simulink model "Fuzzy"  (R2024a)
settings: Solver=VariableStepAuto  StartTime=0.0  StopTime=200  RelTol=1e-3
libraries: fuzblock x1
settings Model: Creator=jyoti  LastModifiedBy=Admin

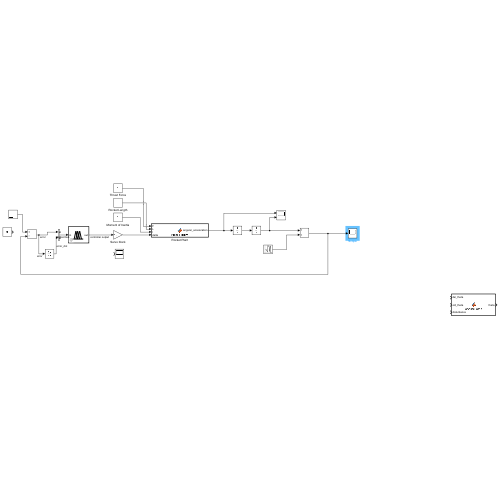
[thumbnail: Simulink's stored preview of the top-level diagram]
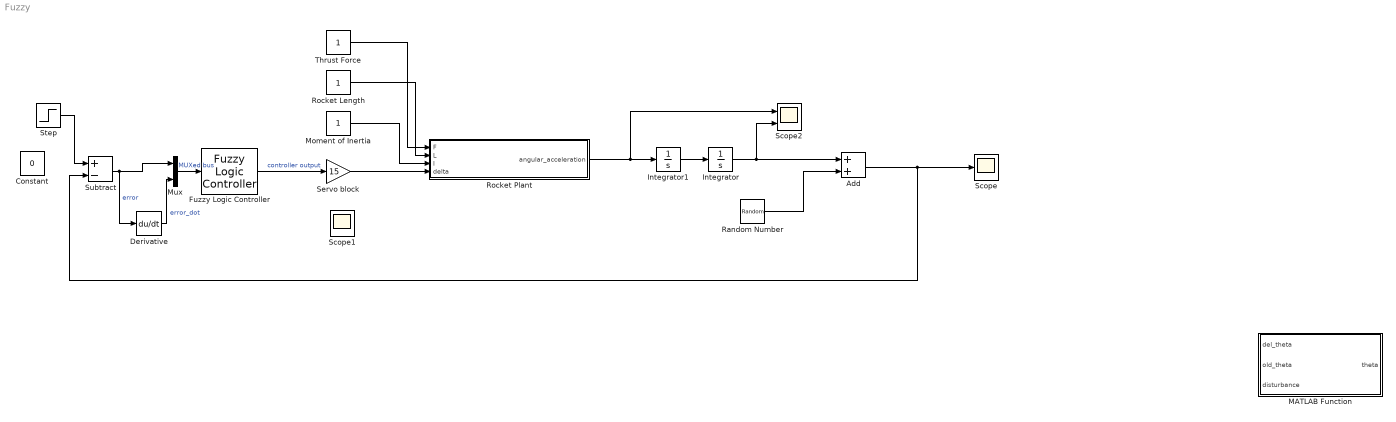
== system Fuzzy ==
  Add : Sum
  Constant : Constant  Value=0
  Derivative : Derivative
  Fuzzy Logic Controller : fuzblock/Fuzzy Logic  Controller  FIS=fis  OutputSampleNumber=101  DataType=double  FuzzifiedInputs=off  RuleFiringStrengths=off  RuleOutputs=off  AggregatedOutputs=off  SimulateUsing=Interpreted execution  OutOfRangeInputValueMessage=warning  NoRuleFiredMessage=warning  EmptyOutputFuzzySetMessage=warning
  Integrator : Integrator
  Integrator1 : Integrator
  MATLAB Function : MATLAB Function  TreatAsAtomicUnit=on
  Moment of Inertia : Constant
  Mux : Mux  Inputs=2
      settings: DisplayOption=signals
  Random Number : RandomNumber  Variance=0.01  SampleTime=0.1
  Rocket Length : Constant
  Rocket Plant : MATLAB Function  TreatAsAtomicUnit=on
  Scope : Scope
  Scope1 : Scope
  Scope2 : Scope  NumInputPorts=2
  Servo block : Gain  Gain=15
  Step : Step  After=8  SampleTime=0
  Subtract : Sum  Inputs=+-
  Thrust Force : Constant
  wires:
  Rocket Length/1 -> Rocket Plant/2(L)
  Moment of Inertia/1 -> Rocket Plant/3(I)
  Thrust Force/1 -> Rocket Plant/1(F)
  Rocket Plant/1(angular_acceleration) -> Integrator1/1, Scope2/1
  Servo block/1 -> Rocket Plant/4(delta)
  Add/1 -> Scope/1, Subtract/2
  Subtract/1 -> Derivative/1, Mux/1  "error"
  Derivative/1 -> Mux/2  "error_dot"
  Fuzzy Logic Controller/1 -> Servo block/1  "controller output"
  Mux/1 -> Fuzzy Logic Controller/1  "MUXed bus"
  Integrator1/1 -> Integrator/1
  Integrator/1 -> Scope2/2, Add/1
  Random Number/1 -> Add/2
  Step/1 -> Subtract/1

== matlab function Fuzzy/MATLAB Function ==
  data: del_theta input; theta output; old_theta input; disturbance input
function theta = accumulator(del_theta, old_theta, disturbance)

theta = old_theta + del_theta + disturbance;

== matlab function Fuzzy/Rocket Plant ==
  data: F input; angular_acceleration output; L input; I input; delta input
function angular_acceleration = rocket_plant(F, L, I, delta)

angular_acceleration = (F*sin(delta)*L)/I;
%omega=  omega+ acc*dt
%theta= theta+ omega*dt
